simulink model "nextpilot_mc_controller"  (R2024b)
settings: configuration reference "ert_windows_generic" (kept outside this file)
settings Model: DataDictionary=nextpilot_datadict.sldd  Creator=CETCA  LastModifiedBy=CETCA
settings ConfigSetRef: SourceName=ert_windows_generic

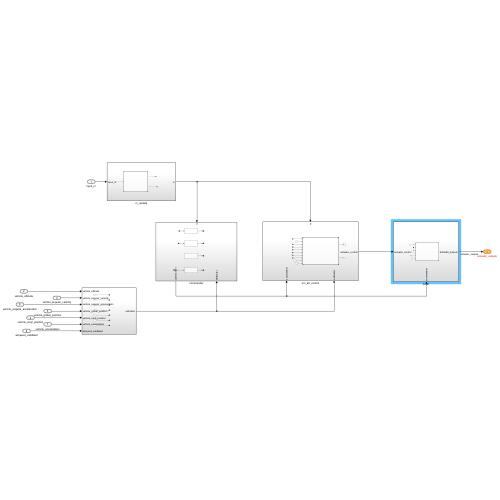
[thumbnail: Simulink's stored preview of the top-level diagram]
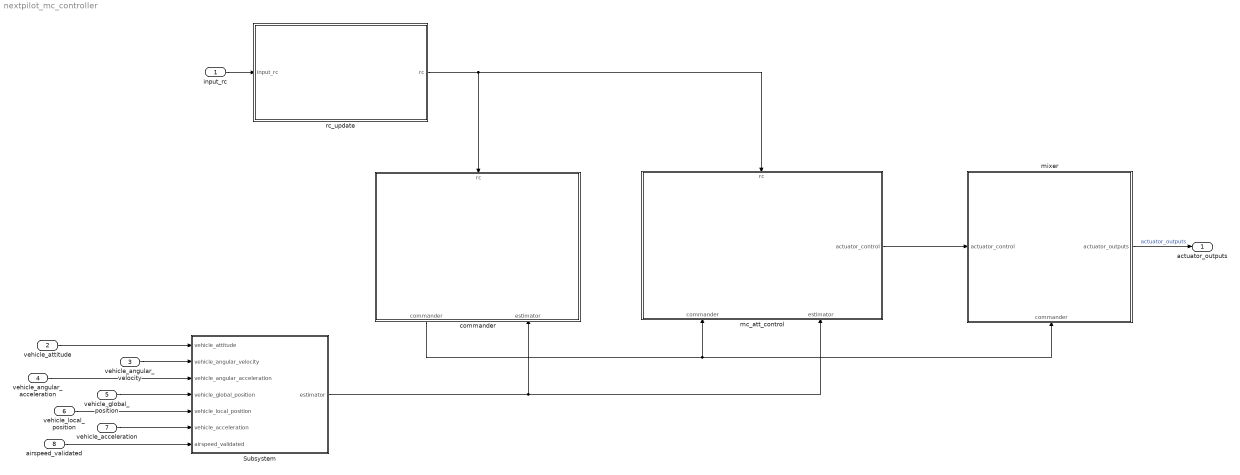
== system nextpilot_mc_controller ==
  input_rc : Inport  OutDataTypeStr=Bus: input_rc_s
  vehicle_attitude : Inport  Port=2  OutDataTypeStr=Bus: vehicle_attitude_s
  vehicle_angular_velocity : Inport  Port=3  OutDataTypeStr=Bus: vehicle_angular_velocity_s
  vehicle_angular_acceleration : Inport  Port=4  OutDataTypeStr=Bus: vehicle_angular_acceleration_s
  vehicle_global_position : Inport  Port=5  OutDataTypeStr=Bus: vehicle_global_position_s
  vehicle_local_position : Inport  Port=6  OutDataTypeStr=Bus: vehicle_local_position_s
  vehicle_acceleration : Inport  Port=7  OutDataTypeStr=Bus: vehicle_acceleration_s
  airspeed_validated : Inport  Port=8  OutDataTypeStr=Bus: airspeed_validated_s
  Subsystem : Subsystem
  commander : Subsystem
      settings: PortSchema="{\"entries\":[{\"content\":{\"sides\":[{\"content\":{},\"type\":\"ConnectorPlacement.EquallySpacedRectSide\",\"uuid\":\"bb59bce1-0500-499a-a754-fb562466c3fb\"},{\"content\":{\"side\":\"RIGHT\"},\"type\":\"ConnectorPlacement.EquallySpacedRectSide\",\"uuid\":\"d03be637-01f7-4508-9bed-614789f3ac84\"},{\"content\":{\"connectorIds\":[\"In1\"],\"side\":\"TOP\"},\"type\":\"ConnectorPlacement.EquallySpacedRectSide\",\"uuid\":\"40f04b52-742b-4cc1-b867-8f89007f8da4\"},{\"content\":{\"connectorIds\":[\"Out1\",\"In2\"],\"side\":\"BOTTOM\"},\"type\":\"ConnectorPlacement.EquallySpacedRectSide\",\"uuid\":\"82adcf13-71aa-4e7e-9e4a-b137b14c20f8\"}]},\"type\":\"ConnectorPlacement.EquallySpacedConnector\",\"uuid\":\"6dab003a-640a-4390-82e5-f1f3e1a9ff99\"}],\"packageUris\":[\"http://schema.mathworks.com/mf0/Connector/R2020b\"],\"version\":\"1.0\"}"
  mc_att_control : Subsystem
      settings: PortSchema="{\"entries\":[{\"content\":{\"sides\":[{\"content\":{},\"type\":\"ConnectorPlacement.EquallySpacedRectSide\",\"uuid\":\"8cc7357a-ade9-4fca-b691-0bf58c66e2d0\"},{\"content\":{\"connectorIds\":[\"Out1\"],\"side\":\"RIGHT\"},\"type\":\"ConnectorPlacement.EquallySpacedRectSide\",\"uuid\":\"b5274986-9954-46fa-b3dc-c31aff903af8\"},{\"content\":{\"connectorIds\":[\"In1\"],\"side\":\"TOP\"},\"type\":\"ConnectorPlacement.EquallySpacedRectSide\",\"uuid\":\"14b6fcf2-4d37-458e-9048-ee99ebe3ce39\"},{\"content\":{\"connectorIds\":[\"In2\",\"In3\"],\"side\":\"BOTTOM\"},\"type\":\"ConnectorPlacement.EquallySpacedRectSide\",\"uuid\":\"af48eb8e-a9e9-4185-b20b-af7f7c9ca0d4\"}]},\"type\":\"ConnectorPlacement.EquallySpacedConnector\",\"uuid\":\"f9df30c3-57ae-4b0b-8783-4331d6574a58\"}],\"packageUris\":[\"http://schema.mathworks.com/mf0/Connector/R2020b\"],\"version\":\"1.0\"}"
  mixer : Subsystem
      settings: PortSchema="{\"entries\":[{\"content\":{\"sides\":[{\"content\":{\"connectorIds\":[\"In1\"]},\"type\":\"ConnectorPlacement.EquallySpacedRectSide\",\"uuid\":\"3d420975-d52f-4ea6-b135-49495d2f3a48\"},{\"content\":{\"connectorIds\":[\"Out1\"],\"side\":\"RIGHT\"},\"type\":\"ConnectorPlacement.EquallySpacedRectSide\",\"uuid\":\"d9c1bfac-a917-4933-9fdf-1d1fd6628fe1\"},{\"content\":{\"side\":\"TOP\"},\"type\":\"ConnectorPlacement.EquallySpacedRectSide\",\"uuid\":\"d6b9a500-1ae7-4512-ba6e-304e74ce2a0b\"},{\"content\":{\"connectorIds\":[\"In2\"],\"side\":\"BOTTOM\"},\"type\":\"ConnectorPlacement.EquallySpacedRectSide\",\"uuid\":\"5a0f04b4-44b8-422f-8a91-088f12e79982\"}]},\"type\":\"ConnectorPlacement.EquallySpacedConnector\",\"uuid\":\"ff4d724c-bb48-4dbc-99a0-795b23573ad3\"}],\"packageUris\":[\"http://schema.mathworks.com/mf0/Connector/R2020b\"],\"version\":\"1.0\"}"
  rc_update : Subsystem
  actuator_outputs : Outport  OutDataTypeStr=Bus: actuator_outputs_s
  wires:
  vehicle_angular_velocity/1 -> Subsystem/2(vehicle_angular_velocity)
  vehicle_acceleration/1 -> Subsystem/6(vehicle_acceleration)
  vehicle_local_position/1 -> Subsystem/5(vehicle_local_position)
  vehicle_global_position/1 -> Subsystem/4(vehicle_global_position)
  vehicle_attitude/1 -> Subsystem/1(vehicle_attitude)
  commander/1(commander) -> mixer/2(commander), mc_att_control/2(commander)
  mixer/1(actuator_outputs) -> actuator_outputs/1  "actuator_outputs"
  mc_att_control/1(actuator_control) -> mixer/1(actuator_control)
  input_rc/1 -> rc_update/1(input_rc)
  rc_update/1(rc) -> mc_att_control/1(rc), commander/1(rc)
  vehicle_angular_acceleration/1 -> Subsystem/3(vehicle_angular_acceleration)
  Subsystem/1(estimator) -> commander/2(estimator), mc_att_control/3(estimator)
  airspeed_validated/1 -> Subsystem/7(airspeed_validated)

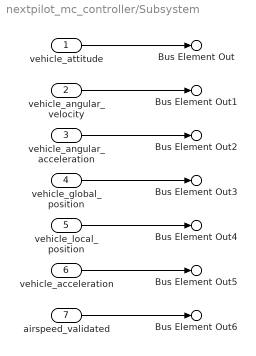
== system nextpilot_mc_controller/Subsystem ==
  vehicle_attitude : Inport
  vehicle_angular_velocity : Inport  Port=2
  vehicle_angular_acceleration : Inport  Port=3
  vehicle_global_position : Inport  Port=4
  vehicle_local_position : Inport  Port=5
  vehicle_acceleration : Inport  Port=6
  airspeed_validated : Inport  Port=7
  Bus Element Out : Outport  PortName=estimator  Element=vehicle_attitude
  Bus Element Out1 : Outport  PortName=estimator  Element=vehicle_angular_velocity
  Bus Element Out2 : Outport  PortName=estimator  Element=vehicle_angular_acceleration
  Bus Element Out3 : Outport  PortName=estimator  Element=vehicle_global_position
  Bus Element Out4 : Outport  PortName=estimator  Element=vehicle_local_position
  Bus Element Out5 : Outport  PortName=estimator  Element=vehicle_acceleration
  Bus Element Out6 : Outport  PortName=estimator  Element=airspeed_validated
  wires:
  vehicle_attitude/1 -> Bus Element Out/1
  vehicle_angular_velocity/1 -> Bus Element Out1/1
  vehicle_angular_acceleration/1 -> Bus Element Out2/1
  vehicle_global_position/1 -> Bus Element Out3/1
  vehicle_local_position/1 -> Bus Element Out4/1
  vehicle_acceleration/1 -> Bus Element Out5/1
  airspeed_validated/1 -> Bus Element Out6/1

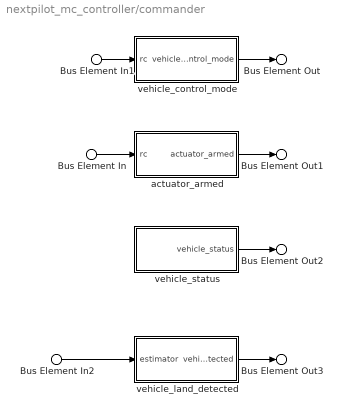
== system nextpilot_mc_controller/commander ==
  Bus Element In : Inport  PortName=rc
  Bus Element In1 : Inport  PortName=rc
  Bus Element In2 : Inport  Port=2  PortName=estimator
  actuator_armed : Subsystem
  vehicle_control_mode : Subsystem
  vehicle_land_detected : Subsystem
  vehicle_status : Subsystem
  Bus Element Out : Outport  PortName=commander  Element=vehicle_control_mode
  Bus Element Out1 : Outport  PortName=commander  Element=actuator_armed
  Bus Element Out2 : Outport  PortName=commander  Element=vehicle_status
  Bus Element Out3 : Outport  PortName=commander  Element=vehicle_land_detected
  wires:
  vehicle_control_mode/1(vehicle_control_mode) -> Bus Element Out/1
  actuator_armed/1(actuator_armed) -> Bus Element Out1/1
  Bus Element In/1 -> actuator_armed/1(rc)
  Bus Element In1/1 -> vehicle_control_mode/1(rc)
  vehicle_status/1(vehicle_status) -> Bus Element Out2/1
  Bus Element In2/1 -> vehicle_land_detected/1(estimator)
  vehicle_land_detected/1(vehicle_land_detected) -> Bus Element Out3/1

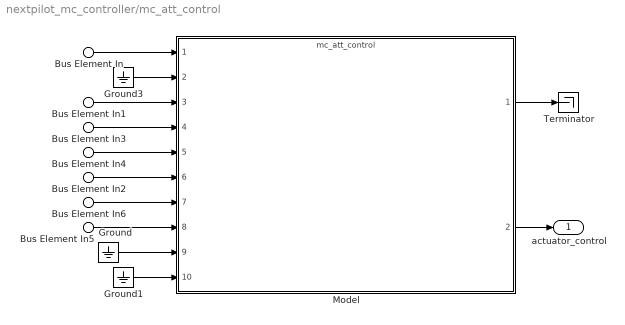
== system nextpilot_mc_controller/mc_att_control ==
  Bus Element In : Inport  PortName=rc  Element=manual_control_setpoint
  Bus Element In2 : Inport  Port=2  PortName=commander  Element=vehicle_control_mode
  Bus Element In5 : Inport  Port=2  PortName=commander  Element=vehicle_land_detected
  Bus Element In6 : Inport  Port=2  PortName=commander  Element=vehicle_status
  Bus Element In1 : Inport  Port=3  PortName=estimator  Element=vehicle_attitude
  Bus Element In3 : Inport  Port=3  PortName=estimator  Element=vehicle_angular_velocity
  Bus Element In4 : Inport  Port=3  PortName=estimator  Element=vehicle_angular_acceleration
  Ground : Ground
  Ground1 : Ground
  Ground3 : Ground
  Model : ModelReference  ModelNameDialog=mc_att_control.slx  SimulationMode=Normal  ModelReferenceVersion=8.95
  Terminator : Terminator
  actuator_control : Outport
  wires:
  Model/1 -> Terminator/1
  Model/2 -> actuator_control/1
  Bus Element In/1 -> Model/1
  Bus Element In3/1 -> Model/4
  Bus Element In1/1 -> Model/3
  Bus Element In2/1 -> Model/6
  Bus Element In6/1 -> Model/7
  Ground3/1 -> Model/2
  Bus Element In4/1 -> Model/5
  Bus Element In5/1 -> Model/8
  Ground/1 -> Model/9
  Ground1/1 -> Model/10

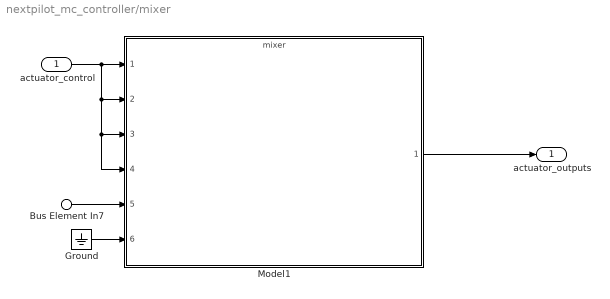
== system nextpilot_mc_controller/mixer ==
  actuator_control : Inport
  Bus Element In7 : Inport  Port=2  PortName=commander  Element=actuator_armed
  Ground : Ground
  Model1 : ModelReference  ModelNameDialog=mixer.slx  SimulationMode=Normal  ModelReferenceVersion=1.81
  actuator_outputs : Outport
  wires:
  Ground/1 -> Model1/6
  Model1/1 -> actuator_outputs/1
  Bus Element In7/1 -> Model1/5
  actuator_control/1 -> Model1/2, Model1/3, Model1/4, Model1/1

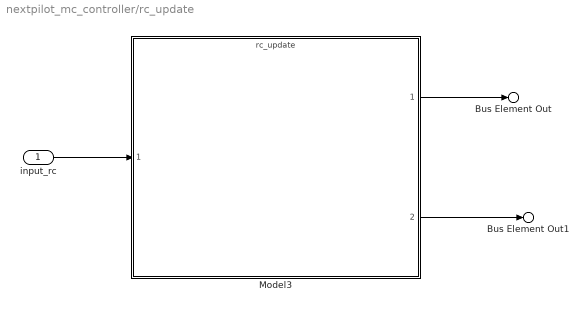
== system nextpilot_mc_controller/rc_update ==
  input_rc : Inport
  Model3 : ModelReference  ModelNameDialog=rc_update.slx  SimulationMode=Normal  ModelReferenceVersion=8.41
  Bus Element Out : Outport  PortName=rc  Element=manual_control_setpoint
  Bus Element Out1 : Outport  PortName=rc  Element=manual_control_switches
  wires:
  Model3/2 -> Bus Element Out1/1
  input_rc/1 -> Model3/1
  Model3/1 -> Bus Element Out/1

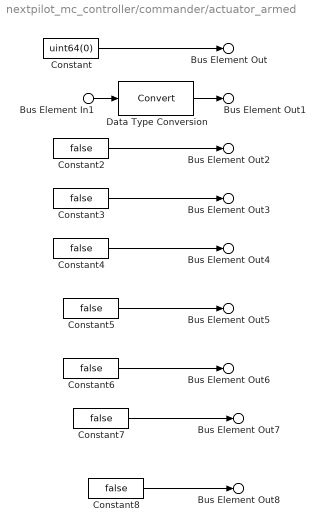
== system nextpilot_mc_controller/commander/actuator_armed ==
  Bus Element In1 : Inport  PortName=rc  Element=manual_control_switches.arm_switch
  Constant : Constant  Value=uint64(0)
  Constant{2..8} (7 alike) : Constant  Value=false
  Data Type Conversion : DataTypeConversion  SaturateOnIntegerOverflow=off  RndMeth=Floor
  Bus Element Out : Outport  PortName=actuator_armed  Element=timestamp
  Bus Element Out1 : Outport  PortName=actuator_armed  Element=armed
  Bus Element Out2 : Outport  PortName=actuator_armed  Element=prearmed
  Bus Element Out3 : Outport  PortName=actuator_armed  Element=ready_to_arm
  Bus Element Out4 : Outport  PortName=actuator_armed  Element=lockdown
  Bus Element Out5 : Outport  PortName=actuator_armed  Element=manual_lockdown
  Bus Element Out6 : Outport  PortName=actuator_armed  Element=force_failsafe
  Bus Element Out7 : Outport  PortName=actuator_armed  Element=in_esc_calibration_mode
  Bus Element Out8 : Outport  PortName=actuator_armed  Element=soft_stop
  wires:
  Constant/1 -> Bus Element Out/1
  Bus Element In1/1 -> Data Type Conversion/1
  Constant2/1 -> Bus Element Out2/1
  Constant3/1 -> Bus Element Out3/1
  Constant4/1 -> Bus Element Out4/1
  Constant5/1 -> Bus Element Out5/1
  Constant6/1 -> Bus Element Out6/1
  Constant7/1 -> Bus Element Out7/1
  Constant8/1 -> Bus Element Out8/1
  Data Type Conversion/1 -> Bus Element Out1/1

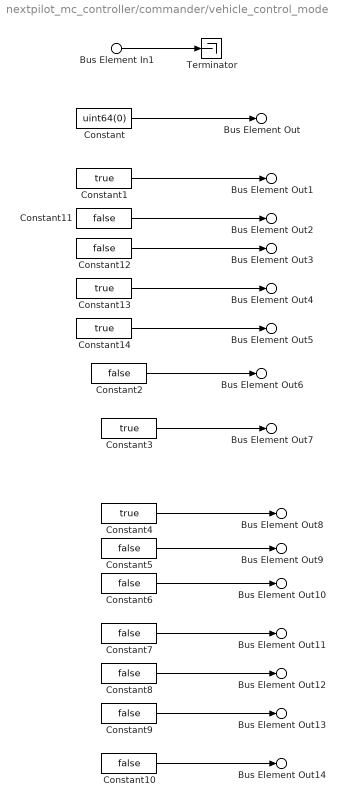
== system nextpilot_mc_controller/commander/vehicle_control_mode ==
  Bus Element In1 : Inport  PortName=rc
  Constant : Constant  Value=uint64(0)
  Constant{1,3..4,13..14} (5 alike) : Constant  Value=true
  Constant{2,5..12} (9 alike) : Constant  Value=false
  Terminator : Terminator
  Bus Element Out : Outport  PortName=vehicle_control_mode  Element=timestamp
  Bus Element Out1 : Outport  PortName=vehicle_control_mode  Element=flag_armed
  Bus Element Out2 : Outport  PortName=vehicle_control_mode  Element=flag_external_manual_override_ok
  Bus Element Out3 : Outport  PortName=vehicle_control_mode  Element=flag_multicopter_position_control_enabled
  Bus Element Out4 : Outport  PortName=vehicle_control_mode  Element=flag_control_manual_enabled
  Bus Element Out5 : Outport  PortName=vehicle_control_mode  Element=flag_control_auto_enabled
  Bus Element Out6 : Outport  PortName=vehicle_control_mode  Element=flag_control_offboard_enabled
  Bus Element Out7 : Outport  PortName=vehicle_control_mode  Element=flag_control_rates_enabled
  Bus Element Out8 : Outport  PortName=vehicle_control_mode  Element=flag_control_attitude_enabled
  Bus Element Out9 : Outport  PortName=vehicle_control_mode  Element=flag_control_acceleration_enabled
  Bus Element Out10 : Outport  PortName=vehicle_control_mode  Element=flag_control_velocity_enabled
  Bus Element Out11 : Outport  PortName=vehicle_control_mode  Element=flag_control_position_enabled
  Bus Element Out12 : Outport  PortName=vehicle_control_mode  Element=flag_control_altitude_enabled
  Bus Element Out13 : Outport  PortName=vehicle_control_mode  Element=flag_control_climb_rate_enabled
  Bus Element Out14 : Outport  PortName=vehicle_control_mode  Element=flag_control_termination_enabled
  wires:
  Constant5/1 -> Bus Element Out9/1
  Constant12/1 -> Bus Element Out3/1
  Constant1/1 -> Bus Element Out1/1
  Constant2/1 -> Bus Element Out6/1
  Constant11/1 -> Bus Element Out2/1
  Constant13/1 -> Bus Element Out4/1
  Constant3/1 -> Bus Element Out7/1
  Constant8/1 -> Bus Element Out12/1
  Constant/1 -> Bus Element Out/1
  Constant14/1 -> Bus Element Out5/1
  Constant9/1 -> Bus Element Out13/1
  Constant10/1 -> Bus Element Out14/1
  Constant7/1 -> Bus Element Out11/1
  Constant6/1 -> Bus Element Out10/1
  Constant4/1 -> Bus Element Out8/1
  Bus Element In1/1 -> Terminator/1

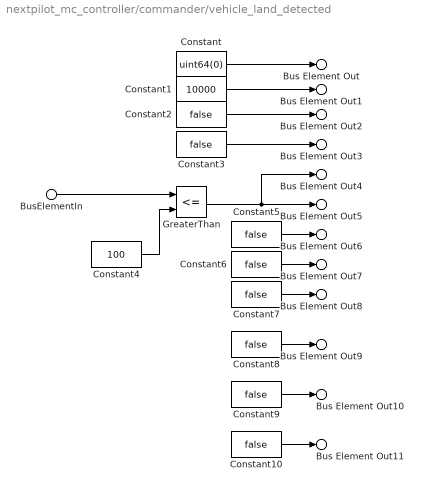
== system nextpilot_mc_controller/commander/vehicle_land_detected ==
  BusElementIn : Inport  PortName=estimator  Element=vehicle_global_position.alt
  Constant : Constant  Value=uint64(0)
  Constant1 : Constant  Value=10000  OutDataTypeStr=single
  Constant{2..3,5..10} (8 alike) : Constant  Value=false
  Constant4 : Constant  Value=100
  GreaterThan : RelationalOperator  Operator=<=  OutDataTypeStr=boolean  RndMeth=Simplest  InputSameDT=off
  Bus Element Out : Outport  PortName=vehicle_land_detected  Element=timestamp
  Bus Element Out1 : Outport  PortName=vehicle_land_detected  Element=alt_max
  Bus Element Out2 : Outport  PortName=vehicle_land_detected  Element=freefall
  Bus Element Out3 : Outport  PortName=vehicle_land_detected  Element=ground_contact
  Bus Element Out4 : Outport  PortName=vehicle_land_detected  Element=maybe_landed
  Bus Element Out5 : Outport  PortName=vehicle_land_detected  Element=landed
  Bus Element Out6 : Outport  PortName=vehicle_land_detected  Element=in_ground_effect
  Bus Element Out7 : Outport  PortName=vehicle_land_detected  Element=in_descend
  Bus Element Out8 : Outport  PortName=vehicle_land_detected  Element=has_low_throttle
  Bus Element Out9 : Outport  PortName=vehicle_land_detected  Element=vertical_movement
  Bus Element Out10 : Outport  PortName=vehicle_land_detected  Element=horizontal_movement
  Bus Element Out11 : Outport  PortName=vehicle_land_detected  Element=close_to_ground_or_skipped_check
  wires:
  Constant/1 -> Bus Element Out/1
  Constant1/1 -> Bus Element Out1/1
  Constant2/1 -> Bus Element Out2/1
  Constant3/1 -> Bus Element Out3/1
  BusElementIn/1 -> GreaterThan/1
  GreaterThan/1 -> Bus Element Out5/1, Bus Element Out4/1
  Constant4/1 -> GreaterThan/2
  Constant5/1 -> Bus Element Out6/1
  Constant6/1 -> Bus Element Out7/1
  Constant7/1 -> Bus Element Out8/1
  Constant9/1 -> Bus Element Out10/1
  Constant10/1 -> Bus Element Out11/1
  Constant8/1 -> Bus Element Out9/1

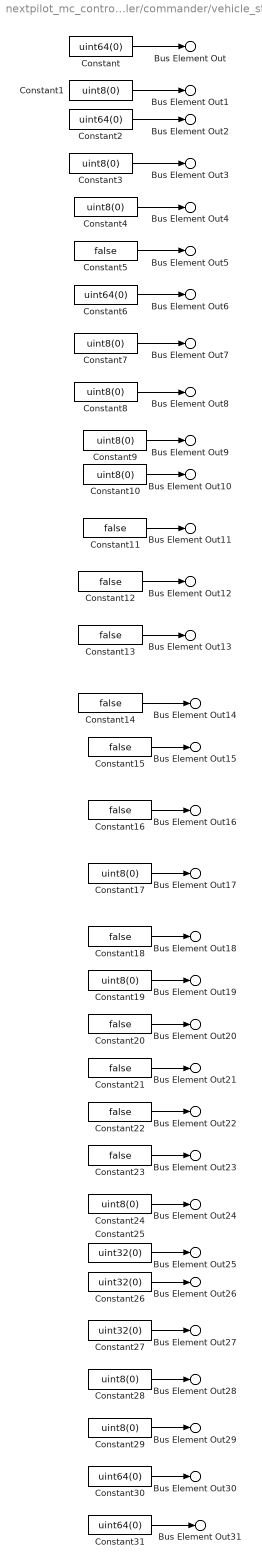
== system nextpilot_mc_controller/commander/vehicle_status ==
  Constant{,2,6,30..31} (5 alike) : Constant  Value=uint64(0)
  Constant{1,3..4,7..10,17,19,24,28..29} (12 alike) : Constant  Value=uint8(0)
  Constant{5,11..16,18,20..23} (12 alike) : Constant  Value=false
  Constant25 : Constant  Value=uint32(0)
  Constant26 : Constant  Value=uint32(0)
  Constant27 : Constant  Value=uint32(0)
  Bus Element Out : Outport  PortName=vehicle_status  Element=timestamp
  Bus Element Out1 : Outport  PortName=vehicle_status  Element=nav_state
  Bus Element Out2 : Outport  PortName=vehicle_status  Element=nav_state_timestamp
  Bus Element Out3 : Outport  PortName=vehicle_status  Element=arming_state
  Bus Element Out4 : Outport  PortName=vehicle_status  Element=hil_state
  Bus Element Out5 : Outport  PortName=vehicle_status  Element=failsafe
  Bus Element Out6 : Outport  PortName=vehicle_status  Element=failsafe_timestamp
  Bus Element Out7 : Outport  PortName=vehicle_status  Element=system_type
  Bus Element Out8 : Outport  PortName=vehicle_status  Element=system_id
  Bus Element Out9 : Outport  PortName=vehicle_status  Element=component_id
  Bus Element Out10 : Outport  PortName=vehicle_status  Element=vehicle_type
  Bus Element Out11 : Outport  PortName=vehicle_status  Element=is_vtol
  Bus Element Out12 : Outport  PortName=vehicle_status  Element=is_vtol_tailsitter
  Bus Element Out13 : Outport  PortName=vehicle_status  Element=vtol_fw_permanent_stab
  Bus Element Out14 : Outport  PortName=vehicle_status  Element=in_transition_mode
  Bus Element Out15 : Outport  PortName=vehicle_status  Element=in_transition_to_fw
  Bus Element Out16 : Outport  PortName=vehicle_status  Element=rc_signal_lost
  Bus Element Out17 : Outport  PortName=vehicle_status  Element=rc_input_mode
  Bus Element Out18 : Outport  PortName=vehicle_status  Element=data_link_lost
  Bus Element Out19 : Outport  PortName=vehicle_status  Element=data_link_lost_counter
  Bus Element Out20 : Outport  PortName=vehicle_status  Element=high_latency_data_link_lost
  Bus Element Out21 : Outport  PortName=vehicle_status  Element=engine_failure
  Bus Element Out22 : Outport  PortName=vehicle_status  Element=mission_failure
  Bus Element Out23 : Outport  PortName=vehicle_status  Element=geofence_violated
  Bus Element Out24 : Outport  PortName=vehicle_status  Element=failure_detector_status
  Bus Element Out25 : Outport  PortName=vehicle_status  Element=onboard_control_sensors_present
  Bus Element Out26 : Outport  PortName=vehicle_status  Element=onboard_control_sensors_enabled
  Bus Element Out27 : Outport  PortName=vehicle_status  Element=onboard_control_sensors_health
  Bus Element Out28 : Outport  PortName=vehicle_status  Element=latest_arming_reason
  Bus Element Out29 : Outport  PortName=vehicle_status  Element=latest_disarming_reason
  Bus Element Out30 : Outport  PortName=vehicle_status  Element=armed_time
  Bus Element Out31 : Outport  PortName=vehicle_status  Element=takeoff_time
  wires:
  Constant/1 -> Bus Element Out/1
  Constant1/1 -> Bus Element Out1/1
  Constant2/1 -> Bus Element Out2/1
  Constant3/1 -> Bus Element Out3/1
  Constant4/1 -> Bus Element Out4/1
  Constant5/1 -> Bus Element Out5/1
  Constant6/1 -> Bus Element Out6/1
  Constant7/1 -> Bus Element Out7/1
  Constant8/1 -> Bus Element Out8/1
  Constant9/1 -> Bus Element Out9/1
  Constant10/1 -> Bus Element Out10/1
  Constant11/1 -> Bus Element Out11/1
  Constant12/1 -> Bus Element Out12/1
  Constant13/1 -> Bus Element Out13/1
  Constant14/1 -> Bus Element Out14/1
  Constant15/1 -> Bus Element Out15/1
  Constant16/1 -> Bus Element Out16/1
  Constant17/1 -> Bus Element Out17/1
  Constant18/1 -> Bus Element Out18/1
  Constant19/1 -> Bus Element Out19/1
  Constant20/1 -> Bus Element Out20/1
  Constant21/1 -> Bus Element Out21/1
  Constant22/1 -> Bus Element Out22/1
  Constant23/1 -> Bus Element Out23/1
  Constant24/1 -> Bus Element Out24/1
  Constant25/1 -> Bus Element Out25/1
  Constant26/1 -> Bus Element Out26/1
  Constant27/1 -> Bus Element Out27/1
  Constant28/1 -> Bus Element Out28/1
  Constant29/1 -> Bus Element Out29/1
  Constant30/1 -> Bus Element Out30/1
  Constant31/1 -> Bus Element Out31/1
